simulink model "PCT_F_Simulink"  (R2024b)
settings: Solver=ode45  StartTime=0.0  StopTime=2  FixedStep=Ts/10000  RelTol=1e-3
values from neighbouring files (symbols this model uses):
  A1 = [-(Rg+Ron)/LM	0;  0 -1/(R*C)]    [Matrici_de_stare.m]    (also in PCT_F.m; PCT_F_magda.m; Pct_A_B_C.m; Pct_D_E.m)
  A2 = [-Rg/(LM*(1+n))	  -1/(LM*(1+n));   1/C	-1/(R*C)]    [Matrici_de_stare.m]    (also in PCT_F.m = [-Rg/(LM*(1+n)^2)	  -1/(LM*(1+n));   1/((1+n)*C)	-1/(R*C)]; PCT_F_magda.m = [-Rg/(LM*(1+ n))	  -1/(LM*(1+n));   1/C	-1/(R*C)]; Pct_A_B_C.m = [-Rg/(LM*(1+n)^2)	  -1/(LM*(1+n));   1/((1+n)*C)	-1/(R*C)]; Pct_D_E.m = [-Rg/(LM*(1+n)^2)	  -1/(LM*(1+n));   1/((1+n)*C)	-1/(R*C)])
  B1 = [1/LM 0;  0  0]    [Matrici_de_stare.m]    (also in PCT_F.m; PCT_F_magda.m; Pct_A_B_C.m; Pct_D_E.m)
  B2 = [1/(LM*(1+n)) -1/(LM*(1+n));  0  0]    [Matrici_de_stare.m]    (also in PCT_F.m; PCT_F_magda.m; Pct_A_B_C.m; Pct_D_E.m)
  D = 0.6    [Matrici_de_stare.m]    (also in PCT_F.m = 0.4599; PCT_F_magda.m = 0.4599; Pct_A_B_C.m = 0.4599; Pct_D_E.m = u)
  F1 = [0 0; 0 0]    [Matrici_de_stare.m]    (also in PCT_F.m; PCT_F_magda.m; Pct_A_B_C.m; Pct_D_E.m)
  F2 = [0 0; 0 0]    [Matrici_de_stare.m]    (also in PCT_F.m; PCT_F_magda.m; Pct_A_B_C.m; Pct_D_E.m)
  Ts = 1/fs    (= 2.5e-05)    [Matrici_de_stare.m]    (also in PCT_F.m; PCT_F_magda.m; Pct_g.m; Pct_g2.m)
  VD = 2.6701    [PCT_F.m]    (also in PCT_F_magda.m = 4.7819; Pct_D_E.m; comutat.m = 0.8; mediat.m = 0.8)
  Vg = 5    [Matrici_de_stare.m]    (also in PCT_F.m; PCT_F_magda.m; Pct_A_B_C.m; Pct_D_E.m)
  X0 = -inv(Ad) * Bd * U    [PCT_F.m]    (also in PCT_F_magda.m)
settings Model: Creator=iorga  LastModifiedBy=iorga

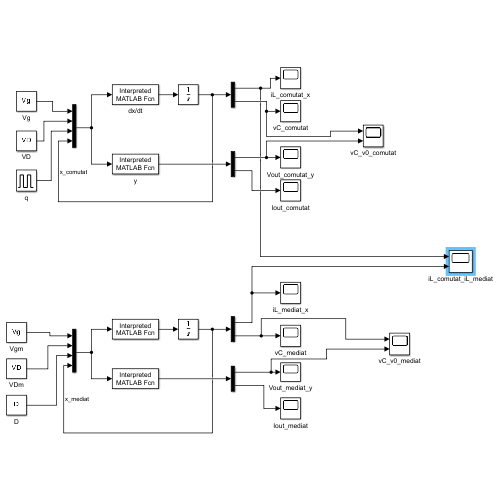
[thumbnail: Simulink's stored preview of the top-level diagram]
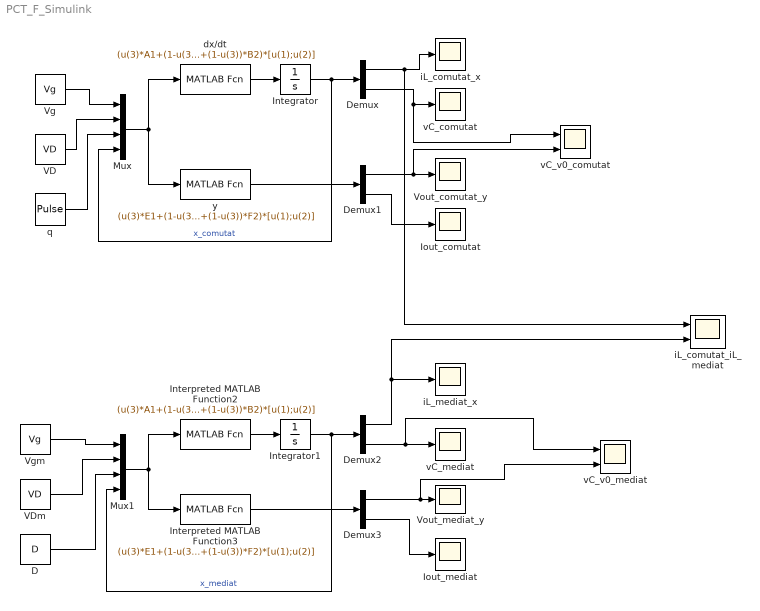
== system PCT_F_Simulink ==
  D : Constant  Value=D
  Demux{,1..3} (4 alike) : Demux  Outputs=2
  Integrator : Integrator  InitialCondition=X0
  Integrator1 : Integrator  InitialCondition=X0
  Interpreted MATLAB Function2 : MATLABFcn  MATLABFcn=(u(3)*A1+(1-u(3))*A2)*[u(4); u(5)]+(u(3)*B1+(1-u(3))*B2)*[u(1);u(2)]  OutputDimensions=2
  Interpreted MATLAB Function3 : MATLABFcn  MATLABFcn=(u(3)*E1+(1-u(3))*E2)*[u(4); u(5)]+(u(3)*F1+(1-u(3))*F2)*[u(1);u(2)]  OutputDimensions=2
  Iout_comutat : Scope
  Iout_mediat : Scope
  Mux : Mux
  Mux1 : Mux
  VD : Constant  Value=VD
  VDm : Constant  Value=VD
  Vg : Constant  Value=Vg
  Vgm : Constant  Value=Vg
  Vout_comutat_y : Scope
  Vout_mediat_y : Scope
  dx/dt : MATLABFcn  MATLABFcn=(u(3)*A1+(1-u(3))*A2)*[u(4); u(5)]+(u(3)*B1+(1-u(3))*B2)*[u(1);u(2)]  OutputDimensions=2
  iL_comutat_iL_mediat : Scope  NumInputPorts=2
  iL_comutat_x : Scope
  iL_mediat_x : Scope
  q : DiscretePulseGenerator  PulseType=Time based  Period=Ts  PulseWidth=D*100
  vC_comutat : Scope
  vC_mediat : Scope
  vC_v0_comutat : Scope  NumInputPorts=2
  vC_v0_mediat : Scope  NumInputPorts=2
  y : MATLABFcn  MATLABFcn=(u(3)*E1+(1-u(3))*E2)*[u(4); u(5)]+(u(3)*F1+(1-u(3))*F2)*[u(1);u(2)]  OutputDimensions=2
  wires:
  D/1 -> Mux1/3
  Demux2/2 -> vC_v0_mediat/1, vC_mediat/1
  q/1 -> Mux/3
  dx/dt/1 -> Integrator/1
  Vg/1 -> Mux/1
  Demux/2 -> vC_v0_comutat/1, vC_comutat/1
  Demux3/1 -> vC_v0_mediat/2, Vout_mediat_y/1
  Interpreted MATLAB Function3/1 -> Demux3/1
  Demux1/1 -> vC_v0_comutat/2, Vout_comutat_y/1
  Interpreted MATLAB Function2/1 -> Integrator1/1
  Demux1/2 -> Iout_comutat/1
  Integrator/1 -> Mux/4, Demux/1  "x_comutat"
  y/1 -> Demux1/1
  Mux1/1 -> Interpreted MATLAB Function2/1, Interpreted MATLAB Function3/1
  Vgm/1 -> Mux1/1
  Mux/1 -> dx/dt/1, y/1
  Demux2/1 -> iL_mediat_x/1, iL_comutat_iL_mediat/2
  VDm/1 -> Mux1/2
  Demux3/2 -> Iout_mediat/1
  Integrator1/1 -> Mux1/4, Demux2/1  "x_mediat"
  VD/1 -> Mux/2
  Demux/1 -> iL_comutat_iL_mediat/1, iL_comutat_x/1
